simulink model "SecondClosedLoop_Final"  (R2018a)
settings: Solver=VariableStepAuto  StartTime=0.0  StopTime=10.0  RelTol=1e-3
values from neighbouring files (symbols this model uses):
  A = [0 0 1 0; 0 0 0 1; 0 -m*g/Mc -Kg^2*Km*Kb/(Mc*Rm*r^2) 0; 0 (Mc+m)*g/(Mc*l) Kg^2*Km*Kb/(Mc*Rm*r^2*l) 0]    [INVERTEDPENDULUM.m]    (also in InvertedPendulum.m)
  B = [0; 0; Km*Kg/(Mc*Rm*r); -Km*Kg/(r*Rm*Mc*l)]    [INVERTEDPENDULUM.m]    (also in InvertedPendulum.m)
  C = eye(4,4)    [INVERTEDPENDULUM.m]    (also in InvertedPendulum.m)
  D = zeros(4,1)    [INVERTEDPENDULUM.m]    (also in InvertedPendulum.m)
  intial_State = [0;0;0;0]    [INVERTEDPENDULUM.m]    (also in InvertedPendulum.m)
  K_alternative = lqr(system_open,Q_alternative,R_alternative)    [InvertedPendulum.m]
  Omega_c = 25*2*pi    (= 157.079632679)    [InvertedPendulum.m]
  reference_State = [1;0;0;0]    [INVERTEDPENDULUM.m]    (also in InvertedPendulum.m = [0;0;0;0])
  T_s = 1/200    (= 0.005)    [InvertedPendulum.m]
  V_max = 5    [InvertedPendulum.m]
libraries: simulink x1
settings Model: Creator=jan  LastModifiedBy=DeKon
settings SFSimCC: SimUseLocalCustomCode=on
settings RTWCC: RTWUseLocalCustomCode=on
settings CodeAppCC: StateflowObjectComments=on

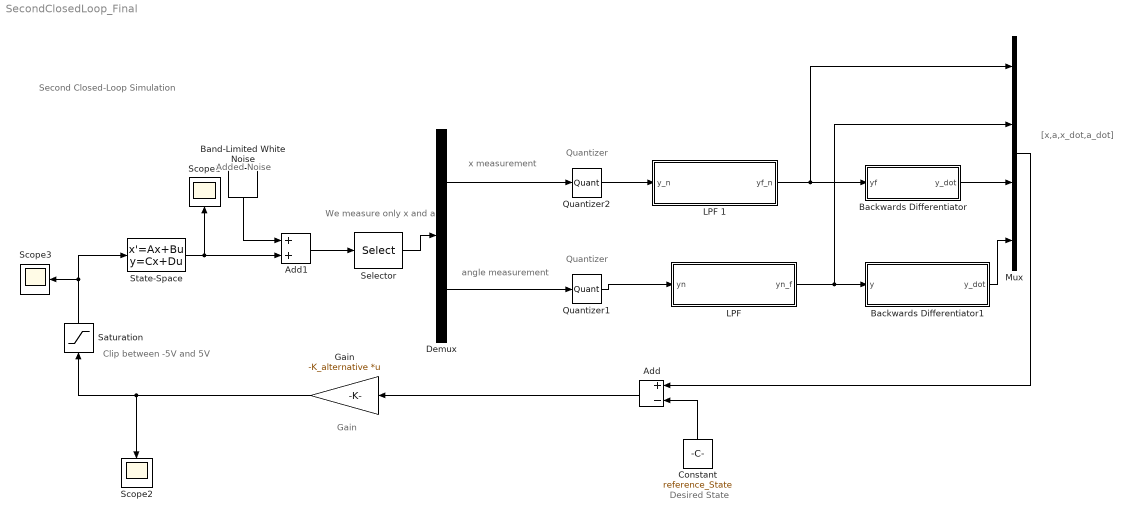
== system SecondClosedLoop_Final ==
  note: Quantizer
  note: Clip between -5V and 5V
  note: Added Noise
  note: Gain
  note: Desired State
  note: Second Closed-Loop Simulation
  note: [x,a,x_dot,a_dot]
  note: angle measurement
  note: x measurement
  note: We measure only x and a
  note: Quantizer
  Add : Sum  Inputs=+-
  Add1 : Sum
  Backwards Differentiator : Subsystem
  Backwards Differentiator1 : Subsystem
  Band-Limited White Noise : simulink/Sources/Band-Limited White Noise  Cov=[10^-8]  Ts=T_s  seed=[23341]
  Constant : Constant  Value=reference_State
  Demux : Demux  Outputs=2
  Gain : Gain  Gain=-K_alternative  Multiplication=Matrix(K*u) (u vector)
  "LPF " : Subsystem
  LPF 1 : Subsystem
  Mux : Mux
  Quantizer1 : Quantizer  QuantizationInterval=Q_interval
  Quantizer2 : Quantizer  QuantizationInterval=Q_interval
  Saturation : Saturate  UpperLimit=V_max  LowerLimit=-V_max
  Scope1 : Scope
  Scope2 : Scope
  Scope3 : Scope
  Selector : Selector  InputPortWidth=4  IndexOptions=Index vector (dialog)  Indices=[1 2]  OutputSizes=1
  State-Space : StateSpace  A=A  B=B  C=C  D=D  InitialCondition=intial_State
  wires:
  Constant/1 -> Add/2
  Add/1 -> Gain/1
  Gain/1 -> Scope2/1, Saturation/1
  Saturation/1 -> Scope3/1, State-Space/1
  Quantizer2/1 -> LPF 1/1(y_n)
  Quantizer1/1 -> "LPF "/1(yn)
  Selector/1 -> Demux/1
  Demux/1 -> Quantizer2/1
  Demux/2 -> Quantizer1/1
  Mux/1 -> Add/1
  "LPF "/1(yn_f) -> Mux/2, Backwards Differentiator1/1(y)
  LPF 1/1(yf_n) -> Mux/1, Backwards Differentiator/1(yf)
  Backwards Differentiator/1(y_dot) -> Mux/3
  Backwards Differentiator1/1(y_dot) -> Mux/4
  Add1/1 -> Selector/1
  State-Space/1 -> Add1/2, Scope1/1
  Band-Limited White Noise/1 -> Add1/1

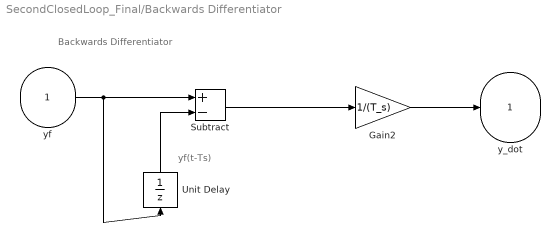
== system SecondClosedLoop_Final/Backwards Differentiator ==
  note: yf(t-Ts)
  note: Backwards Differentiator
  yf : Inport
  Gain2 : Gain  Gain=1/(T_s)
  Subtract : Sum  Inputs=+-
  Unit Delay : UnitDelay  SampleTime=T_s
  y_dot : Outport
  wires:
  yf/1 -> Unit Delay/1, Subtract/1
  Unit Delay/1 -> Subtract/2
  Subtract/1 -> Gain2/1
  Gain2/1 -> y_dot/1

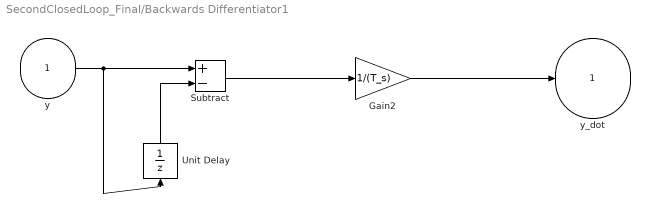
== system SecondClosedLoop_Final/Backwards Differentiator1 ==
  y : Inport
  Gain2 : Gain  Gain=1/(T_s)
  Subtract : Sum  Inputs=+-
  Unit Delay : UnitDelay  SampleTime=T_s
  y_dot : Outport
  wires:
  Gain2/1 -> y_dot/1
  Subtract/1 -> Gain2/1
  Unit Delay/1 -> Subtract/2
  y/1 -> Subtract/1, Unit Delay/1

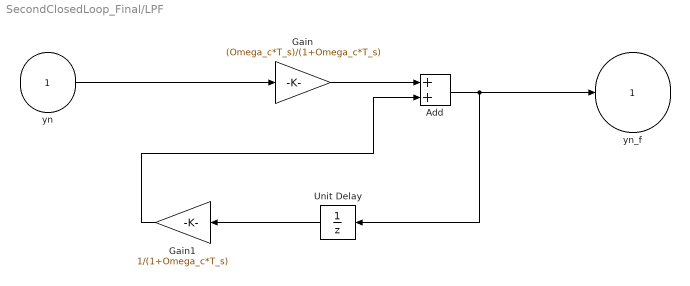
== system SecondClosedLoop_Final/LPF  ==
  yn : Inport
  Add : Sum
  Gain : Gain  Gain=(Omega_c*T_s)/(1+Omega_c*T_s)
  Gain1 : Gain  Gain=1/(1+Omega_c*T_s)
  Unit Delay : UnitDelay  SampleTime=T_s
  yn_f : Outport
  wires:
  Gain1/1 -> Add/2
  Add/1 -> Unit Delay/1, yn_f/1
  Gain/1 -> Add/1
  Unit Delay/1 -> Gain1/1
  yn/1 -> Gain/1

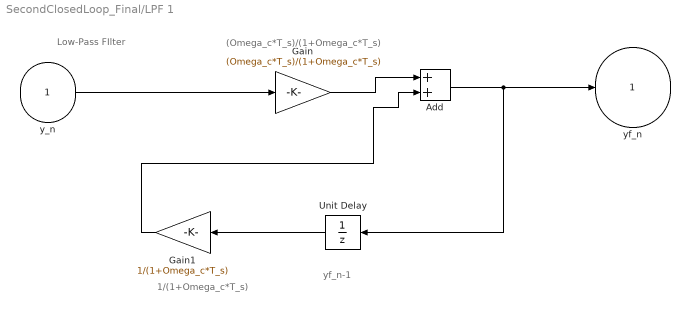
== system SecondClosedLoop_Final/LPF 1 ==
  note: Low-Pass FIlter
  note: yf_n-1
  note: 1/(1+Omega_c*T_s)
  note: (Omega_c*T_s)/(1+Omega_c*T_s)
  y_n : Inport
  Add : Sum
  Gain : Gain  Gain=(Omega_c*T_s)/(1+Omega_c*T_s)
  Gain1 : Gain  Gain=1/(1+Omega_c*T_s)
  Unit Delay : UnitDelay  SampleTime=T_s
  yf_n : Outport
  wires:
  y_n/1 -> Gain/1
  Unit Delay/1 -> Gain1/1
  Gain/1 -> Add/1
  Add/1 -> Unit Delay/1, yf_n/1
  Gain1/1 -> Add/2
